simulink model "IEEE9Buses"  (R2024b)
settings: Solver=FixedStepAuto  StartTime=0  StopTime=5  FixedStep=1e-6  RelTol=1e-3
values from neighbouring files (symbols this model uses):
  SG_D_1_D = 0.01056    [SG9_parameters.m]
  SG_D_1_EnableSaturation = 0    [SG9_parameters.m]
  SG_D_1_f0 = 60    [SG9_parameters.m]
  SG_D_1_H = 7.5    [SG9_parameters.m]
  SG_D_1_K_A = 20    [SG9_parameters.m]
  SG_D_1_K_E = 1.000000e+1    (= 10)    [SG9_parameters.m]
  SG_D_1_K_F = 2.363    [SG9_parameters.m]
  SG_D_1_K_s = 5    [SG9_parameters.m]
  SG_D_1_R_a = 0.001088    [SG9_parameters.m]
  SG_D_1_S_A = 1    [SG9_parameters.m]
  SG_D_1_S_B = 0.103    [SG9_parameters.m]
  SG_D_1_S_N = 10.659857    [SG9_parameters.m]
  SG_D_1_SpeedPara = 200    [SG9_parameters.m]
  SG_D_1_T_0 = 0.720173    [SG9_parameters.m]
  SG_D_1_T_1 = 0.3    [SG9_parameters.m]
  SG_D_1_T_2 = 0.05    [SG9_parameters.m]
  SG_D_1_T_3 = 0.02    [SG9_parameters.m]
  SG_D_1_T_4 = 0.005    [SG9_parameters.m]
  SG_D_1_T_A = 0.02    [SG9_parameters.m]
  SG_D_1_T_dd = 8.000000e+0    (= 8)    [SG9_parameters.m]
  SG_D_1_T_ddd = 0.04    [SG9_parameters.m]
  SG_D_1_T_E = 0.314    [SG9_parameters.m]
  SG_D_1_T_F = 0.35    [SG9_parameters.m]
  SG_D_1_T_qd = 0.8    [SG9_parameters.m]
  SG_D_1_T_qdd = 0.02    [SG9_parameters.m]
  SG_D_1_T_speed = 0.1    [SG9_parameters.m]
  SG_D_1_T_w = 0.5    [SG9_parameters.m]
  SG_D_1_V_ref = 1.990276    [SG9_parameters.m]
  SG_D_1_w_ref = 376.991118    [SG9_parameters.m]
  SG_D_1_x_d = 1.9    [SG9_parameters.m]
  SG_D_1_x_dd = 0.302    [SG9_parameters.m]
  SG_D_1_x_ddd = 0.204    [SG9_parameters.m]
  SG_D_1_x_l = 0.05    [SG9_parameters.m]
  SG_D_1_x_q = 1.3    [SG9_parameters.m]
  SG_D_1_x_qd = 0.5    [SG9_parameters.m]
  SG_D_1_x_qdd = 0.3    [SG9_parameters.m]
  SG_D_2_D = 0.01056    [SG9_parameters.m]
  SG_D_2_EnableSaturation = 0    [SG9_parameters.m]
  SG_D_2_f0 = 60    [SG9_parameters.m]
  SG_D_2_H = 7.5    [SG9_parameters.m]
  SG_D_2_K_A = 20    [SG9_parameters.m]
  SG_D_2_K_E = 1.000000e+1    (= 10)    [SG9_parameters.m]
  SG_D_2_K_F = 2.363    [SG9_parameters.m]
  SG_D_2_K_s = 0.5    [SG9_parameters.m]
  SG_D_2_R_a = 0.001088    [SG9_parameters.m]
  SG_D_2_S_A = 1    [SG9_parameters.m]
  SG_D_2_S_B = 0.103    [SG9_parameters.m]
  SG_D_2_S_N = 10.659857    [SG9_parameters.m]
  SG_D_2_SpeedPara = 200    [SG9_parameters.m]
  SG_D_2_T_0 = 1.632913    [SG9_parameters.m]
  SG_D_2_T_1 = 0.2    [SG9_parameters.m]
  SG_D_2_T_2 = 0.05    [SG9_parameters.m]
  SG_D_2_T_3 = 0.02    [SG9_parameters.m]
  SG_D_2_T_4 = 0.005    [SG9_parameters.m]
  SG_D_2_T_A = 0.02    [SG9_parameters.m]
  SG_D_2_T_dd = 8.000000e+0    (= 8)    [SG9_parameters.m]
  SG_D_2_T_ddd = 0.04    [SG9_parameters.m]
  SG_D_2_T_E = 0.314    [SG9_parameters.m]
  SG_D_2_T_F = 0.35    [SG9_parameters.m]
  SG_D_2_T_qd = 0.8    [SG9_parameters.m]
  SG_D_2_T_qdd = 0.02    [SG9_parameters.m]
  SG_D_2_T_speed = 0.1    [SG9_parameters.m]
  SG_D_2_T_w = 0.5    [SG9_parameters.m]
  SG_D_2_V_ref = 2.662631    [SG9_parameters.m]
  SG_D_2_w_ref = 376.991118    [SG9_parameters.m]
  SG_D_2_x_d = 1.9    [SG9_parameters.m]
  SG_D_2_x_dd = 0.302    [SG9_parameters.m]
  SG_D_2_x_ddd = 0.204    [SG9_parameters.m]
  SG_D_2_x_l = 0.05    [SG9_parameters.m]
  SG_D_2_x_q = 1.3    [SG9_parameters.m]
  SG_D_2_x_qd = 0.5    [SG9_parameters.m]
  SG_D_2_x_qdd = 0.3    [SG9_parameters.m]
  SG_D_3_D = 0.01056    [SG9_parameters.m]
  SG_D_3_EnableSaturation = 0    [SG9_parameters.m]
  SG_D_3_f0 = 60    [SG9_parameters.m]
  SG_D_3_H = 7.5    [SG9_parameters.m]
  SG_D_3_K_A = 20    [SG9_parameters.m]
  SG_D_3_K_E = 1.000000e+1    (= 10)    [SG9_parameters.m]
  SG_D_3_K_F = 2.363    [SG9_parameters.m]
  SG_D_3_K_s = 0.5    [SG9_parameters.m]
  SG_D_3_R_a = 0.001088    [SG9_parameters.m]
  SG_D_3_S_A = 1    [SG9_parameters.m]
  SG_D_3_S_B = 0.103    [SG9_parameters.m]
  SG_D_3_S_N = 10.659857    [SG9_parameters.m]
  SG_D_3_SpeedPara = 200    [SG9_parameters.m]
  SG_D_3_T_0 = 0.850788    [SG9_parameters.m]
  SG_D_3_T_1 = 0.2    [SG9_parameters.m]
  SG_D_3_T_2 = 0.05    [SG9_parameters.m]
  SG_D_3_T_3 = 0.02    [SG9_parameters.m]
  SG_D_3_T_4 = 0.005    [SG9_parameters.m]
  SG_D_3_T_A = 0.02    [SG9_parameters.m]
  SG_D_3_T_dd = 8.000000e+0    (= 8)    [SG9_parameters.m]
  SG_D_3_T_ddd = 0.04    [SG9_parameters.m]
  SG_D_3_T_E = 0.314    [SG9_parameters.m]
  SG_D_3_T_F = 0.35    [SG9_parameters.m]
  SG_D_3_T_qd = 0.8    [SG9_parameters.m]
  SG_D_3_T_qdd = 0.02    [SG9_parameters.m]
  SG_D_3_T_speed = 0.1    [SG9_parameters.m]
  SG_D_3_T_w = 0.5    [SG9_parameters.m]
  SG_D_3_V_ref = 1.915682    [SG9_parameters.m]
  SG_D_3_w_ref = 376.991118    [SG9_parameters.m]
  SG_D_3_x_d = 1.9    [SG9_parameters.m]
  SG_D_3_x_dd = 0.302    [SG9_parameters.m]
  SG_D_3_x_ddd = 0.204    [SG9_parameters.m]
  SG_D_3_x_l = 0.05    [SG9_parameters.m]
  SG_D_3_x_q = 1.3    [SG9_parameters.m]
  SG_D_3_x_qd = 0.5    [SG9_parameters.m]
  SG_D_3_x_qdd = 0.3    [SG9_parameters.m]
(part 1 of 9)
settings Model: SimulationMode=accelerator  Creator=Greg  LastModifiedBy=Greg
settings DataIOCC: ReturnWorkspaceOutputs=off

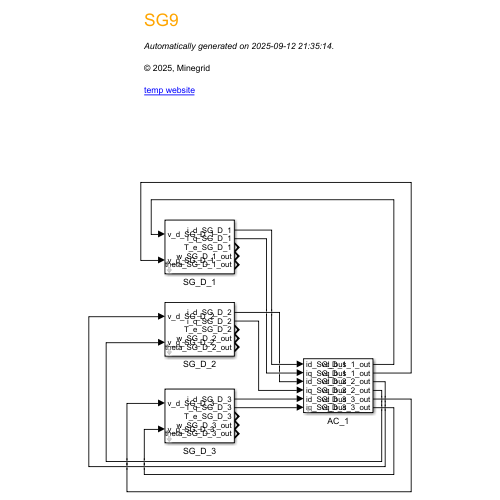
[thumbnail: Simulink's stored preview of the top-level diagram]
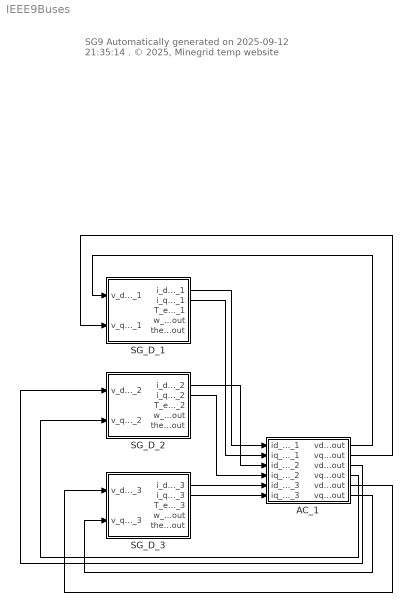
== system IEEE9Buses ==
  note: SG9
      | Automatically generated on 2025-09-12 21:35:14 .
      | © 2025, Minegrid
      | temp website
  AC_1 : Subsystem  mask(AC_1){}
      mask help: Parameters Interface of AC_1
  SG_D_1 : Subsystem  mask(SG_D_1){T_0=SG_D_1_T_0, w_ref=SG_D_1_w_ref, V_ref=SG_D_1_V_ref, x_d=SG_D_1_x_d, x_dd=SG_D_1_x_dd, x_ddd=SG_D_1_x_ddd, x_q=SG_D_1_x_q, x_qd=SG_D_1_x_qd, x_qdd=SG_D_1_x_qdd, x_l=SG_D_1_x_l, R_a=SG_D_1_R_a, T_dd=SG_D_1_T_dd, T_ddd=SG_D_1_T_ddd, T_qd=SG_D_1_T_qd, T_qdd=SG_D_1_T_qdd, H=SG_D_1_H, D=SG_D_1_D, SpeedPara=SG_D_1_SpeedPara, K_A=SG_D_1_K_A, EnableSaturation=SG_D_1_EnableSaturation, f0=SG_D_1_f0, T_speed=SG_D_1_T_speed, T_E=SG_D_1_T_E, T_A=SG_D_1_T_A, T_F=SG_D_1_T_F, K_E=SG_D_1_K_E, K_F=SG_D_1_K_F, K_s=SG_D_1_K_s, T_1=SG_D_1_T_1, T_2=SG_D_1_T_2, T_3=SG_D_1_T_3, T_4=SG_D_1_T_4, T_w=SG_D_1_T_w, S_A=SG_D_1_S_A, S_B=SG_D_1_S_B, S_N=SG_D_1_S_N}
      mask help: Parameters Interface of SG_D_1
  SG_D_2 : Subsystem  mask(SG_D_2){T_0=SG_D_2_T_0, w_ref=SG_D_2_w_ref, V_ref=SG_D_2_V_ref, x_d=SG_D_2_x_d, x_dd=SG_D_2_x_dd, x_ddd=SG_D_2_x_ddd, x_q=SG_D_2_x_q, x_qd=SG_D_2_x_qd, x_qdd=SG_D_2_x_qdd, x_l=SG_D_2_x_l, R_a=SG_D_2_R_a, T_dd=SG_D_2_T_dd, T_ddd=SG_D_2_T_ddd, T_qd=SG_D_2_T_qd, T_qdd=SG_D_2_T_qdd, H=SG_D_2_H, D=SG_D_2_D, SpeedPara=SG_D_2_SpeedPara, K_A=SG_D_2_K_A, EnableSaturation=SG_D_2_EnableSaturation, f0=SG_D_2_f0, T_speed=SG_D_2_T_speed, T_E=SG_D_2_T_E, T_A=SG_D_2_T_A, T_F=SG_D_2_T_F, K_E=SG_D_2_K_E, K_F=SG_D_2_K_F, K_s=SG_D_2_K_s, T_1=SG_D_2_T_1, T_2=SG_D_2_T_2, T_3=SG_D_2_T_3, T_4=SG_D_2_T_4, T_w=SG_D_2_T_w, S_A=SG_D_2_S_A, S_B=SG_D_2_S_B, S_N=SG_D_2_S_N}
      mask help: Parameters Interface of SG_D_2
  SG_D_3 : Subsystem  mask(SG_D_3){T_0=SG_D_3_T_0, w_ref=SG_D_3_w_ref, V_ref=SG_D_3_V_ref, x_d=SG_D_3_x_d, x_dd=SG_D_3_x_dd, x_ddd=SG_D_3_x_ddd, x_q=SG_D_3_x_q, x_qd=SG_D_3_x_qd, x_qdd=SG_D_3_x_qdd, x_l=SG_D_3_x_l, R_a=SG_D_3_R_a, T_dd=SG_D_3_T_dd, T_ddd=SG_D_3_T_ddd, T_qd=SG_D_3_T_qd, T_qdd=SG_D_3_T_qdd, H=SG_D_3_H, D=SG_D_3_D, SpeedPara=SG_D_3_SpeedPara, K_A=SG_D_3_K_A, EnableSaturation=SG_D_3_EnableSaturation, f0=SG_D_3_f0, T_speed=SG_D_3_T_speed, T_E=SG_D_3_T_E, T_A=SG_D_3_T_A, T_F=SG_D_3_T_F, K_E=SG_D_3_K_E, K_F=SG_D_3_K_F, K_s=SG_D_3_K_s, T_1=SG_D_3_T_1, T_2=SG_D_3_T_2, T_3=SG_D_3_T_3, T_4=SG_D_3_T_4, T_w=SG_D_3_T_w, S_A=SG_D_3_S_A, S_B=SG_D_3_S_B, S_N=SG_D_3_S_N}
      mask help: Parameters Interface of SG_D_3
  wires:
  SG_D_2/2(i_q_SG_D_2) -> AC_1/4(iq_SG_D_2)
  SG_D_1/2(i_q_SG_D_1) -> AC_1/2(iq_SG_D_1)
  SG_D_1/1(i_d_SG_D_1) -> AC_1/1(id_SG_D_1)
  SG_D_2/1(i_d_SG_D_2) -> AC_1/3(id_SG_D_2)
  AC_1/1(vd_bus_1_out) -> SG_D_1/1(v_d_SG_D_1)
  SG_D_3/1(i_d_SG_D_3) -> AC_1/5(id_SG_D_3)
  AC_1/2(vq_bus_1_out) -> SG_D_1/2(v_q_SG_D_1)
  SG_D_3/2(i_q_SG_D_3) -> AC_1/6(iq_SG_D_3)
  AC_1/3(vd_bus_2_out) -> SG_D_2/1(v_d_SG_D_2)
  AC_1/4(vq_bus_2_out) -> SG_D_2/2(v_q_SG_D_2)
  AC_1/5(vd_bus_3_out) -> SG_D_3/1(v_d_SG_D_3)
  AC_1/6(vq_bus_3_out) -> SG_D_3/2(v_q_SG_D_3)

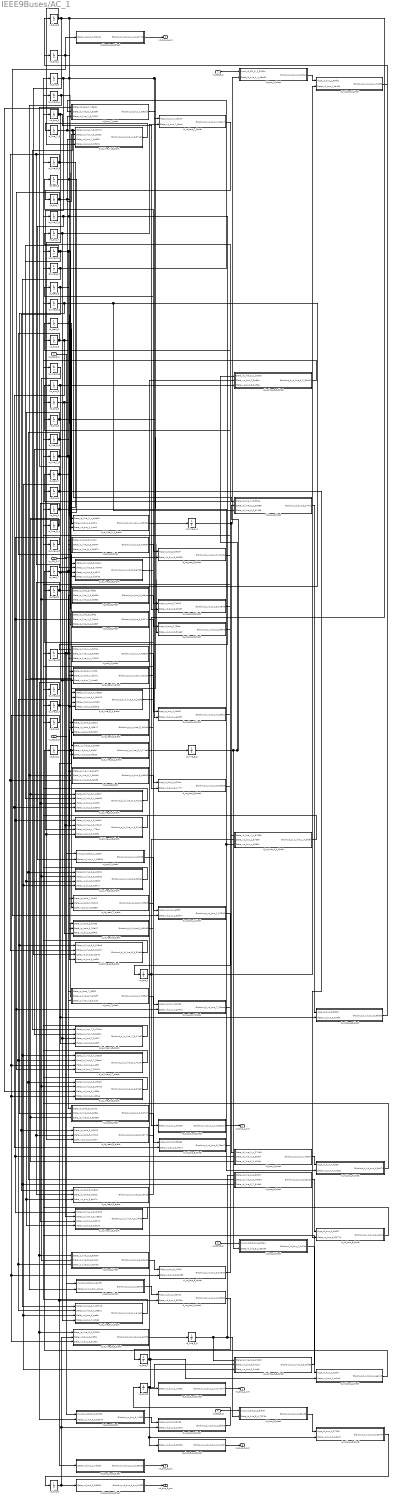
== system IEEE9Buses/AC_1 ==
  id_SG_D_1 : Inport
  iq_SG_D_1 : Inport  Port=2
  id_SG_D_2 : Inport  Port=3
  iq_SG_D_2 : Inport  Port=4
  id_SG_D_3 : Inport  Port=5
  iq_SG_D_3 : Inport  Port=6
  d_id_line_1_4_block : Subsystem
  d_id_line_3_6_block : Subsystem
  d_id_line_4_5_block : Subsystem
  d_id_line_5_6_block : Subsystem
  d_id_line_6_7_block : Subsystem
  d_id_line_7_8_block : Subsystem
  d_id_line_8_2_block : Subsystem
  d_id_line_8_9_block : Subsystem
  d_id_line_9_4_block : Subsystem
  d_id_load_5_block : Subsystem
  d_id_load_7_block : Subsystem
  d_id_load_9_block : Subsystem
  d_iq_line_1_4_block : Subsystem
  d_iq_line_3_6_block : Subsystem
  d_iq_line_4_5_block : Subsystem
  d_iq_line_5_6_block : Subsystem
  d_iq_line_6_7_block : Subsystem
  d_iq_line_7_8_block : Subsystem
  d_iq_line_8_2_block : Subsystem
  d_iq_line_8_9_block : Subsystem
  d_iq_line_9_4_block : Subsystem
  d_iq_load_5_block : Subsystem
  d_iq_load_7_block : Subsystem
  d_iq_load_9_block : Subsystem
  d_vd_bus_1_block : Subsystem
  d_vd_bus_2_block : Subsystem
  d_vd_bus_3_block : Subsystem
  d_vd_bus_4_block : Subsystem
  d_vd_bus_5_block : Subsystem
  d_vd_bus_6_block : Subsystem
  d_vd_bus_7_block : Subsystem
  d_vd_bus_8_block : Subsystem
  d_vd_bus_9_block : Subsystem
  d_vq_bus_1_block : Subsystem
  d_vq_bus_2_block : Subsystem
  d_vq_bus_3_block : Subsystem
  d_vq_bus_4_block : Subsystem
  d_vq_bus_5_block : Subsystem
  d_vq_bus_6_block : Subsystem
  d_vq_bus_7_block : Subsystem
  d_vq_bus_8_block : Subsystem
  d_vq_bus_9_block : Subsystem
  id_bus_1_block : Subsystem
  id_bus_2_block : Subsystem
  id_bus_3_block : Subsystem
  id_bus_4_block : Subsystem
  id_bus_5_block : Subsystem
  id_bus_6_block : Subsystem
  id_bus_7_block : Subsystem
  id_bus_8_block : Subsystem
  id_bus_9_block : Subsystem
  id_line_1_4 : Integrator  InitialCondition=0.7195
  id_line_3_6 : Integrator  InitialCondition=0.844
  id_line_4_5 : Integrator  InitialCondition=0.308
  id_line_5_6 : Integrator  InitialCondition=-0.6084
  id_line_6_7 : Integrator  InitialCondition=0.2452
  id_line_7_8 : Integrator  InitialCondition=-0.7713
  id_line_8_2 : Integrator  InitialCondition=-1.6311
  id_line_8_9 : Integrator  InitialCondition=0.8749
  id_line_9_4 : Integrator  InitialCondition=-0.4046
  id_load_5 : Integrator  InitialCondition=0.898817607082261
  id_load_7 : Integrator  InitialCondition=1.0183565162188208
  id_load_9 : Integrator  InitialCondition=1.2619557605717109
  iq_bus_1_block : Subsystem
  iq_bus_2_block : Subsystem
  iq_bus_3_block : Subsystem
  iq_bus_4_block : Subsystem
  iq_bus_5_block : Subsystem
  iq_bus_6_block : Subsystem
  iq_bus_7_block : Subsystem
  iq_bus_8_block : Subsystem
  iq_bus_9_block : Subsystem
  iq_line_1_4 : Integrator  InitialCondition=-0.2407
  iq_line_3_6 : Integrator  InitialCondition=0.1071
  iq_line_4_5 : Integrator  InitialCondition=-0.085
  iq_line_5_6 : Integrator  InitialCondition=0.0353
  iq_line_6_7 : Integrator  InitialCondition=-0.1419
  iq_line_7_8 : Integrator  InitialCondition=0.0257
  iq_line_8_2 : Integrator  InitialCondition=-0.1312
  iq_line_8_9 : Integrator  InitialCondition=-0.0692
  iq_line_9_4 : Integrator  InitialCondition=0.3203
  iq_load_5 : Integrator  InitialCondition=-0.37142447893959263
  iq_load_7 : Integrator  InitialCondition=-0.34407079769452764
  iq_load_9 : Integrator  InitialCondition=-0.6196286093512099
  vd_bus_1 : Integrator  InitialCondition=1.0
  vd_bus_1_out_block : Subsystem
  vd_bus_2 : Integrator  InitialCondition=0.9857952451733694
  vd_bus_2_out_block : Subsystem
  vd_bus_3 : Integrator  InitialCondition=0.9965349784480291
  vd_bus_3_out_block : Subsystem
  vd_bus_4 : Integrator  InitialCondition=0.9861362779327475
  vd_bus_5 : Integrator  InitialCondition=0.9730754311923555
  vd_bus_6 : Integrator  InitialCondition=1.0028088352065478
  vd_bus_7 : Integrator  InitialCondition=0.9855868856760395
  vd_bus_8 : Integrator  InitialCondition=0.9939961188157862
  vd_bus_9 : Integrator  InitialCondition=0.9548625268660215
  vq_bus_1 : Integrator  InitialCondition=0.0
  vq_bus_1_out_block : Subsystem
  vq_bus_2 : Integrator  InitialCondition=0.16795158407581826
  vq_bus_2_out_block : Subsystem
  vq_bus_3 : Integrator  InitialCondition=0.08317473612573835
  vq_bus_3_out_block : Subsystem
  vq_bus_4 : Integrator  InitialCondition=-0.04144590802322367
  vq_bus_5 : Integrator  InitialCondition=-0.06833870911689703
  vq_bus_6 : Integrator  InitialCondition=0.03371518392178962
  vq_bus_7 : Integrator  InitialCondition=0.01069206498389038
  vq_bus_8 : Integrator  InitialCondition=0.06600581865802534
  vq_bus_9 : Integrator  InitialCondition=-0.07263340166698863
  vd_bus_1_out : Outport
  vq_bus_1_out : Outport  Port=2
  vd_bus_2_out : Outport  Port=3
  vq_bus_2_out : Outport  Port=4
  vd_bus_3_out : Outport  Port=5
  vq_bus_3_out : Outport  Port=6
  wires:
  d_vd_bus_8_block/1(Blockout_d_vd_bus_8_9b000) -> vd_bus_8/1
  iq_bus_2_block/1(Blockout_iq_bus_2_e5997) -> d_vq_bus_2_block/1(Alge_iq_bus_2_d512d)
  vd_bus_6/1 -> d_vq_bus_6_block/2(State_vd_bus_6_b0c85), d_id_line_3_6_block/3(State_vd_bus_6_a239d), d_id_line_5_6_block/4(State_vd_bus_6_469ee), d_id_line_6_7_block/3(State_vd_bus_6_443fc)
  iq_bus_9_block/1(Blockout_iq_bus_9_40080) -> d_vq_bus_9_block/1(Alge_iq_bus_9_d9c5f)
  id_bus_3_block/1(Blockout_id_bus_3_8623b) -> d_vd_bus_3_block/1(Alge_id_bus_3_37259)
  id_bus_8_block/1(Blockout_id_bus_8_27f10) -> d_vd_bus_8_block/1(Alge_id_bus_8_fc0d0)
  d_id_line_1_4_block/1(Blockout_d_id_line_1_4_93c8d) -> id_line_1_4/1
  vq_bus_2_out_block/1(Blockout_vq_bus_2_out_74947) -> vq_bus_2_out/1
  iq_SG_D_3/1 -> iq_bus_3_block/1(Input_iq_SG_D_3_d199a)
  vd_bus_3_out_block/1(Blockout_vd_bus_3_out_02f53) -> vd_bus_3_out/1
  d_iq_line_8_2_block/1(Blockout_d_iq_line_8_2_3b9b1) -> iq_line_8_2/1
  d_vd_bus_4_block/1(Blockout_d_vd_bus_4_3a074) -> vd_bus_4/1
  id_SG_D_3/1 -> id_bus_3_block/1(Input_id_SG_D_3_5cb67)
  id_SG_D_2/1 -> id_bus_2_block/1(Input_id_SG_D_2_e59e4)
  iq_SG_D_2/1 -> iq_bus_2_block/1(Input_iq_SG_D_2_644f3)
  iq_SG_D_1/1 -> iq_bus_1_block/1(Input_iq_SG_D_1_ca28f)
  id_bus_9_block/1(Blockout_id_bus_9_52737) -> d_vd_bus_9_block/1(Alge_id_bus_9_59e86)
  d_vd_bus_3_block/1(Blockout_d_vd_bus_3_60d94) -> vd_bus_3/1
  vq_bus_9/1 -> d_vd_bus_9_block/2(State_vq_bus_9_f7872), d_iq_line_9_4_block/4(State_vq_bus_9_ae56d), d_iq_load_9_block/3(State_vq_bus_9_5d2b3), d_iq_line_8_9_block/4(State_vq_bus_9_bbb4a)
  d_vq_bus_6_block/1(Blockout_d_vq_bus_6_6730a) -> vq_bus_6/1
  id_SG_D_1/1 -> id_bus_1_block/1(Input_id_SG_D_1_3262c)
  d_id_line_3_6_block/1(Blockout_d_id_line_3_6_e09c3) -> id_line_3_6/1
  d_vq_bus_5_block/1(Blockout_d_vq_bus_5_a48d8) -> vq_bus_5/1
  vq_bus_3_out_block/1(Blockout_vq_bus_3_out_11dc3) -> vq_bus_3_out/1
  iq_bus_8_block/1(Blockout_iq_bus_8_e3563) -> d_vq_bus_8_block/1(Alge_iq_bus_8_c37e6)
  iq_bus_7_block/1(Blockout_iq_bus_7_33867) -> d_vq_bus_7_block/1(Alge_iq_bus_7_d2b8e)
  vd_bus_1/1 -> d_id_line_1_4_block/2(State_vd_bus_1_adf11), vd_bus_1_out_block/1(State_vd_bus_1_30b4d), d_vq_bus_1_block/2(State_vd_bus_1_09d77)
  iq_line_8_9/1 -> d_id_line_8_9_block/2(State_iq_line_8_9_9c429), iq_bus_8_block/3(State_iq_line_8_9_ce938), d_iq_line_8_9_block/2(State_iq_line_8_9_4d480), iq_bus_9_block/2(State_iq_line_8_9_c4804)
  id_bus_7_block/1(Blockout_id_bus_7_881bd) -> d_vd_bus_7_block/1(Alge_id_bus_7_c3139)
  id_bus_5_block/1(Blockout_id_bus_5_5017c) -> d_vd_bus_5_block/1(Alge_id_bus_5_7f9ce)
  iq_bus_6_block/1(Blockout_iq_bus_6_e51e3) -> d_vq_bus_6_block/1(Alge_iq_bus_6_c7a6f)
  d_id_load_7_block/1(Blockout_d_id_load_7_5535f) -> id_load_7/1
  vd_bus_7/1 -> d_id_load_7_block/3(State_vd_bus_7_a9ee9), d_id_line_7_8_block/3(State_vd_bus_7_ec582), d_vq_bus_7_block/2(State_vd_bus_7_25076), d_id_line_6_7_block/4(State_vd_bus_7_82461)
  d_id_load_9_block/1(Blockout_d_id_load_9_d90d0) -> id_load_9/1
  id_line_8_9/1 -> d_id_line_8_9_block/1(State_id_line_8_9_b15e6), id_bus_9_block/2(State_id_line_8_9_2ef8e), id_bus_8_block/3(State_id_line_8_9_87c38), d_iq_line_8_9_block/1(State_id_line_8_9_9ac4c)
  iq_line_6_7/1 -> iq_bus_6_block/3(State_iq_line_6_7_0570d), d_iq_line_6_7_block/2(State_iq_line_6_7_68911), d_id_line_6_7_block/2(State_iq_line_6_7_95ec9), iq_bus_7_block/2(State_iq_line_6_7_a92f3)
  id_line_4_5/1 -> d_iq_line_4_5_block/1(State_id_line_4_5_bb2d8), id_bus_4_block/2(State_id_line_4_5_666cf), d_id_line_4_5_block/1(State_id_line_4_5_9d9bf), id_bus_5_block/2(State_id_line_4_5_7fba6)
  id_bus_6_block/1(Blockout_id_bus_6_b82c2) -> d_vd_bus_6_block/1(Alge_id_bus_6_00f20)
  iq_bus_5_block/1(Blockout_iq_bus_5_cd3aa) -> d_vq_bus_5_block/1(Alge_iq_bus_5_7cd16)
  id_bus_2_block/1(Blockout_id_bus_2_0c7b0) -> d_vd_bus_2_block/1(Alge_id_bus_2_43cf4)
  id_line_6_7/1 -> id_bus_6_block/3(State_id_line_6_7_545c3), d_iq_line_6_7_block/1(State_id_line_6_7_95748), d_id_line_6_7_block/1(State_id_line_6_7_a6336), id_bus_7_block/2(State_id_line_6_7_e269f)
  iq_bus_4_block/1(Blockout_iq_bus_4_66e6a) -> d_vq_bus_4_block/1(Alge_iq_bus_4_4be37)
  d_vq_bus_9_block/1(Blockout_d_vq_bus_9_7a2cb) -> vq_bus_9/1
  iq_line_9_4/1 -> iq_bus_4_block/3(State_iq_line_9_4_7b513), iq_bus_9_block/3(State_iq_line_9_4_0e87b), d_iq_line_9_4_block/2(State_iq_line_9_4_5ae9b), d_id_line_9_4_block/2(State_iq_line_9_4_9b423)
  vq_bus_6/1 -> d_iq_line_6_7_block/3(State_vq_bus_6_aeffa), d_iq_line_3_6_block/3(State_vq_bus_6_14cd6), d_iq_line_5_6_block/4(State_vq_bus_6_e6417), d_vd_bus_6_block/2(State_vq_bus_6_6b77a)
  id_load_5/1 -> d_iq_load_5_block/1(State_id_load_5_3469a), d_id_load_5_block/1(State_id_load_5_6942d), id_bus_5_block/1(State_id_load_5_1fb8c)
  iq_bus_3_block/1(Blockout_iq_bus_3_7a5f4) -> d_vq_bus_3_block/1(Alge_iq_bus_3_4618e)
  id_line_5_6/1 -> d_id_line_5_6_block/1(State_id_line_5_6_30ca9), id_bus_6_block/2(State_id_line_5_6_48a69), d_iq_line_5_6_block/1(State_id_line_5_6_bb5d1), id_bus_5_block/3(State_id_line_5_6_0d80f)
  id_bus_4_block/1(Blockout_id_bus_4_7eb34) -> d_vd_bus_4_block/1(Alge_id_bus_4_fcb80)
  vd_bus_1_out_block/1(Blockout_vd_bus_1_out_0277b) -> vd_bus_1_out/1
  vq_bus_1_out_block/1(Blockout_vq_bus_1_out_8292c) -> vq_bus_1_out/1
  id_line_9_4/1 -> id_bus_4_block/3(State_id_line_9_4_46c2c), id_bus_9_block/3(State_id_line_9_4_80368), d_iq_line_9_4_block/1(State_id_line_9_4_069c7), d_id_line_9_4_block/1(State_id_line_9_4_75390)
  iq_line_8_2/1 -> iq_bus_2_block/2(State_iq_line_8_2_4a7a6), iq_bus_8_block/2(State_iq_line_8_2_9e1b5), d_id_line_8_2_block/1(State_iq_line_8_2_d048e)
  iq_bus_1_block/1(Blockout_iq_bus_1_b29d9) -> d_vq_bus_1_block/1(Alge_iq_bus_1_ef3c8)
  id_bus_1_block/1(Blockout_id_bus_1_d304c) -> d_vd_bus_1_block/1(Alge_id_bus_1_5efe2)
  vd_bus_2_out_block/1(Blockout_vd_bus_2_out_05523) -> vd_bus_2_out/1
  d_id_line_8_2_block/1(Blockout_d_id_line_8_2_17ce9) -> id_line_8_2/1
  vq_bus_5/1 -> d_iq_load_5_block/3(State_vq_bus_5_8a47c), d_iq_line_4_5_block/4(State_vq_bus_5_6d109), d_iq_line_5_6_block/3(State_vq_bus_5_5a835), d_vd_bus_5_block/2(State_vq_bus_5_81ea0)
  d_id_line_9_4_block/1(Blockout_d_id_line_9_4_bcdf8) -> id_line_9_4/1
  vd_bus_8/1 -> d_vq_bus_8_block/2(State_vd_bus_8_17777), d_id_line_8_2_block/3(State_vd_bus_8_4faee), d_id_line_8_9_block/3(State_vd_bus_8_2da45), d_id_line_7_8_block/4(State_vd_bus_8_932d1)
  iq_load_5/1 -> d_iq_load_5_block/2(State_iq_load_5_30dc2), d_id_load_5_block/2(State_iq_load_5_374bd), iq_bus_5_block/1(State_iq_load_5_4f98c)
  id_load_7/1 -> d_iq_load_7_block/1(State_id_load_7_27cc0), d_id_load_7_block/1(State_id_load_7_9c11f), id_bus_7_block/1(State_id_load_7_766eb)
  id_line_8_2/1 -> d_iq_line_8_2_block/1(State_id_line_8_2_1a8da), id_bus_8_block/2(State_id_line_8_2_3b688), id_bus_2_block/2(State_id_line_8_2_6326a)
  id_line_3_6/1 -> id_bus_3_block/2(State_id_line_3_6_7876d), id_bus_6_block/1(State_id_line_3_6_8987c), d_iq_line_3_6_block/1(State_id_line_3_6_232a9)
  iq_line_7_8/1 -> iq_bus_7_block/3(State_iq_line_7_8_2c1c0), iq_bus_8_block/1(State_iq_line_7_8_aee75), d_id_line_7_8_block/2(State_iq_line_7_8_ca362), d_iq_line_7_8_block/2(State_iq_line_7_8_5efa1)
  id_line_7_8/1 -> d_id_line_7_8_block/1(State_id_line_7_8_3b707), d_iq_line_7_8_block/1(State_id_line_7_8_521a4), id_bus_8_block/1(State_id_line_7_8_ffd1a), id_bus_7_block/3(State_id_line_7_8_76347)
  vd_bus_2/1 -> d_vq_bus_2_block/2(State_vd_bus_2_9829a), vd_bus_2_out_block/1(State_vd_bus_2_7ad9e), d_id_line_8_2_block/2(State_vd_bus_2_bbfdf)
  iq_line_3_6/1 -> d_id_line_3_6_block/1(State_iq_line_3_6_282d0), iq_bus_3_block/2(State_iq_line_3_6_8aa40), iq_bus_6_block/1(State_iq_line_3_6_58a90)
  iq_line_5_6/1 -> d_id_line_5_6_block/2(State_iq_line_5_6_587be), iq_bus_6_block/2(State_iq_line_5_6_012cd), d_iq_line_5_6_block/2(State_iq_line_5_6_03d26), iq_bus_5_block/3(State_iq_line_5_6_de832)
  iq_line_4_5/1 -> d_id_line_4_5_block/2(State_iq_line_4_5_254e7), d_iq_line_4_5_block/2(State_iq_line_4_5_78e2b), iq_bus_4_block/2(State_iq_line_4_5_eba88), iq_bus_5_block/2(State_iq_line_4_5_8b006)
  iq_load_7/1 -> d_id_load_7_block/2(State_iq_load_7_51219), d_iq_load_7_block/2(State_iq_load_7_db75c), iq_bus_7_block/1(State_iq_load_7_0f831)
  id_line_1_4/1 -> id_bus_1_block/2(State_id_line_1_4_5eb51), id_bus_4_block/1(State_id_line_1_4_271d8), d_iq_line_1_4_block/1(State_id_line_1_4_57d80)
  vq_bus_4/1 -> d_iq_line_1_4_block/3(State_vq_bus_4_b5984), d_vd_bus_4_block/2(State_vq_bus_4_57d81), d_iq_line_9_4_block/3(State_vq_bus_4_81c39), d_iq_line_4_5_block/3(State_vq_bus_4_a5b76)
  iq_line_1_4/1 -> d_id_line_1_4_block/1(State_iq_line_1_4_a5e26), iq_bus_4_block/1(State_iq_line_1_4_f419e), iq_bus_1_block/2(State_iq_line_1_4_8883d)
  vd_bus_4/1 -> d_vq_bus_4_block/2(State_vd_bus_4_edd2f), d_id_line_9_4_block/3(State_vd_bus_4_e2c56), d_id_line_1_4_block/3(State_vd_bus_4_44d4f), d_id_line_4_5_block/3(State_vd_bus_4_779cd)
  iq_load_9/1 -> d_id_load_9_block/2(State_iq_load_9_20a57), d_iq_load_9_block/2(State_iq_load_9_d6a72), iq_bus_9_block/1(State_iq_load_9_c7d1b)
  vq_bus_1/1 -> d_vd_bus_1_block/2(State_vq_bus_1_fa40c), d_iq_line_1_4_block/2(State_vq_bus_1_b7ee6), vq_bus_1_out_block/1(State_vq_bus_1_02b5e)
  id_load_9/1 -> d_id_load_9_block/1(State_id_load_9_f793a), d_iq_load_9_block/1(State_id_load_9_2692c), id_bus_9_block/1(State_id_load_9_21730)
  vd_bus_5/1 -> d_id_line_4_5_block/4(State_vd_bus_5_5d0f4), d_id_load_5_block/3(State_vd_bus_5_7ebb7), d_vq_bus_5_block/2(State_vd_bus_5_232bf), d_id_line_5_6_block/3(State_vd_bus_5_135fa)
  vd_bus_9/1 -> d_id_line_8_9_block/4(State_vd_bus_9_bcf84), d_id_line_9_4_block/4(State_vd_bus_9_f9bbb), d_vq_bus_9_block/2(State_vd_bus_9_b3036), d_id_load_9_block/3(State_vd_bus_9_d8fb5)
  vq_bus_8/1 -> d_vd_bus_8_block/2(State_vq_bus_8_879f9), d_iq_line_7_8_block/4(State_vq_bus_8_ca51f), d_iq_line_8_9_block/3(State_vq_bus_8_a4521), d_iq_line_8_2_block/3(State_vq_bus_8_54d3e)
  vq_bus_7/1 -> d_iq_line_6_7_block/4(State_vq_bus_7_cc662), d_iq_line_7_8_block/3(State_vq_bus_7_5101f), d_iq_load_7_block/3(State_vq_bus_7_44ad8), d_vd_bus_7_block/2(State_vq_bus_7_fddcc)
  vd_bus_3/1 -> d_vq_bus_3_block/2(State_vd_bus_3_13373), d_id_line_3_6_block/2(State_vd_bus_3_4df94), vd_bus_3_out_block/1(State_vd_bus_3_69656)
  vq_bus_3/1 -> d_vd_bus_3_block/2(State_vq_bus_3_a84ef), vq_bus_3_out_block/1(State_vq_bus_3_9203b), d_iq_line_3_6_block/2(State_vq_bus_3_b412d)
  vq_bus_2/1 -> d_vd_bus_2_block/2(State_vq_bus_2_cc1ad), vq_bus_2_out_block/1(State_vq_bus_2_14eae), d_iq_line_8_2_block/2(State_vq_bus_2_6a8ad)
  d_vq_bus_1_block/1(Blockout_d_vq_bus_1_67500) -> vq_bus_1/1
  d_id_line_7_8_block/1(Blockout_d_id_line_7_8_9746d) -> id_line_7_8/1
  d_id_line_6_7_block/1(Blockout_d_id_line_6_7_75140) -> id_line_6_7/1
  d_iq_line_6_7_block/1(Blockout_d_iq_line_6_7_a4a1a) -> iq_line_6_7/1
  d_iq_load_5_block/1(Blockout_d_iq_load_5_26519) -> iq_load_5/1
  d_id_line_5_6_block/1(Blockout_d_id_line_5_6_0d6a1) -> id_line_5_6/1
  d_id_line_4_5_block/1(Blockout_d_id_line_4_5_01c13) -> id_line_4_5/1
  d_id_line_8_9_block/1(Blockout_d_id_line_8_9_50e3a) -> id_line_8_9/1
  d_vq_bus_3_block/1(Blockout_d_vq_bus_3_efd63) -> vq_bus_3/1
  d_id_load_5_block/1(Blockout_d_id_load_5_1877c) -> id_load_5/1
  d_vq_bus_4_block/1(Blockout_d_vq_bus_4_2eed2) -> vq_bus_4/1
  d_iq_line_1_4_block/1(Blockout_d_iq_line_1_4_afc5f) -> iq_line_1_4/1
  d_iq_line_3_6_block/1(Blockout_d_iq_line_3_6_9df33) -> iq_line_3_6/1
  d_vq_bus_7_block/1(Blockout_d_vq_bus_7_29dea) -> vq_bus_7/1
  d_iq_line_4_5_block/1(Blockout_d_iq_line_4_5_7f0d8) -> iq_line_4_5/1
  d_iq_line_5_6_block/1(Blockout_d_iq_line_5_6_f65e1) -> iq_line_5_6/1
  d_iq_load_9_block/1(Blockout_d_iq_load_9_040c9) -> iq_load_9/1
  d_iq_line_7_8_block/1(Blockout_d_iq_line_7_8_47c62) -> iq_line_7_8/1
  d_vd_bus_2_block/1(Blockout_d_vd_bus_2_ea113) -> vd_bus_2/1
  d_iq_line_8_9_block/1(Blockout_d_iq_line_8_9_a326a) -> iq_line_8_9/1
  d_iq_line_9_4_block/1(Blockout_d_iq_line_9_4_42bd3) -> iq_line_9_4/1
  d_iq_load_7_block/1(Blockout_d_iq_load_7_b1dc5) -> iq_load_7/1
  d_vq_bus_8_block/1(Blockout_d_vq_bus_8_0c63e) -> vq_bus_8/1
  d_vd_bus_1_block/1(Blockout_d_vd_bus_1_31f38) -> vd_bus_1/1
  d_vd_bus_9_block/1(Blockout_d_vd_bus_9_33aa7) -> vd_bus_9/1
  d_vd_bus_5_block/1(Blockout_d_vd_bus_5_ffea6) -> vd_bus_5/1
  d_vd_bus_7_block/1(Blockout_d_vd_bus_7_02e17) -> vd_bus_7/1
  d_vd_bus_6_block/1(Blockout_d_vd_bus_6_a81cc) -> vd_bus_6/1
  d_vq_bus_2_block/1(Blockout_d_vq_bus_2_b988a) -> vq_bus_2/1

== system IEEE9Buses/SG_D_1 ==
  v_d_SG_D_1 : Inport
  v_q_SG_D_1 : Inport  Port=2
  E_fd_SG_D_1 : Integrator  InitialCondition=1.9805513012329263
  Px_1_SG_D_1 : Integrator  InitialCondition=0.0
  Px_2_SG_D_1 : Integrator  InitialCondition=0.0
  Px_3_SG_D_1 : Integrator  InitialCondition=1.3587350977693559e-31
  R_f_SG_D_1 : Integrator  InitialCondition=13.371550642324015
  T_e_SG_D_1_block : Subsystem
  T_m_SG_D_1 : Integrator  InitialCondition=0.7201733550664303
  V_f_SG_D_1 : Integrator  InitialCondition=19.805513012329264
  d_E_fd_SG_D_1_block : Subsystem
  d_Px_1_SG_D_1_block : Subsystem
  d_Px_2_SG_D_1_block : Subsystem
  d_Px_3_SG_D_1_block : Subsystem
  d_R_f_SG_D_1_block : Subsystem
  d_T_m_SG_D_1_block : Subsystem
  d_V_f_SG_D_1_block : Subsystem
  d_psi_1d_SG_D_1_block : Subsystem
  d_psi_d_SG_D_1_block : Subsystem
  d_psi_fd_SG_D_1_block : Subsystem
  d_psi_gq_SG_D_1_block : Subsystem
  d_psi_kq_SG_D_1_block : Subsystem
  d_psi_q_SG_D_1_block : Subsystem
  d_theta_SG_D_1_block : Subsystem
  d_w_SG_D_1_block : Subsystem
  i_d_SG_D_1_block : Subsystem
  i_q_SG_D_1_block : Subsystem
  psi_1d_SG_D_1 : Integrator  InitialCondition=0.845823229911384
  psi_d_SG_D_1 : Integrator  InitialCondition=0.8151549036594502
  psi_fd_SG_D_1 : Integrator  InitialCondition=1.0003915942211292
  psi_gq_SG_D_1 : Integrator  InitialCondition=0.35728835356649113
  psi_kq_SG_D_1 : Integrator  InitialCondition=-0.5582630524476424
  psi_q_SG_D_1 : Integrator  InitialCondition=-0.580593574545548
  theta_SG_D_1 : Integrator  InitialCondition=0.6186381378069596
  theta_SG_D_1_out_block : Subsystem
  w_SG_D_1 : Integrator  InitialCondition=376.99111843077515
  w_SG_D_1_out_block : Subsystem
  i_d_SG_D_1 : Outport
  i_q_SG_D_1 : Outport  Port=2
  T_e_SG_D_1 : Outport  Port=3
  w_SG_D_1_out : Outport  Port=4
  theta_SG_D_1_out : Outport  Port=5
  wires:
  d_Px_1_SG_D_1_block/1(Blockout_d_Px_1_SG_D_1_cf474) -> Px_1_SG_D_1/1
  V_f_SG_D_1/1 -> d_V_f_SG_D_1_block/14(State_V_f_SG_D_1_8970f), d_E_fd_SG_D_1_block/2(State_V_f_SG_D_1_23896)
  psi_kq_SG_D_1/1 -> d_psi_q_SG_D_1_block/2(State_psi_kq_SG_D_1_3d8c9), d_V_f_SG_D_1_block/10(State_psi_kq_SG_D_1_48f93), d_w_SG_D_1_block/5(State_psi_kq_SG_D_1_49621), i_d_SG_D_1_block/2(State_psi_kq_SG_D_1_e3ffd), i_q_SG_D_1_block/2(State_psi_kq_SG_D_1_bbf34), d_psi_kq_SG_D_1_block/4(State_psi_kq_SG_D_1_6f435), d_psi_kq_SG_D_1_block/2(State_psi_kq_SG_D_1_2245f), d_psi_gq_SG_D_1_block/3(State_psi_kq_SG_D_1_536d2), d_psi_gq_SG_D_1_block/5(State_psi_kq_SG_D_1_a18e9), d_psi_gq_SG_D_1_block/8(State_psi_kq_SG_D_1_64214), T_e_SG_D_1_block/3(State_psi_kq_SG_D_1_b55ca)
  w_SG_D_1_out_block/1(Blockout_w_SG_D_1_out_88950) -> w_SG_D_1_out/1
  d_theta_SG_D_1_block/1(Blockout_d_theta_SG_D_1_2b5f4) -> theta_SG_D_1/1
  w_SG_D_1/1 -> d_Px_2_SG_D_1_block/4(State_w_SG_D_1_fc7e0), d_Px_1_SG_D_1_block/2(State_w_SG_D_1_abb95), d_psi_d_SG_D_1_block/9(State_w_SG_D_1_13bdb), d_w_SG_D_1_block/1(State_w_SG_D_1_f41ee), d_T_m_SG_D_1_block/1(State_w_SG_D_1_aacae), d_V_f_SG_D_1_block/8(State_w_SG_D_1_1fa23), d_theta_SG_D_1_block/1(State_w_SG_D_1_e3939), d_V_f_SG_D_1_block/13(State_w_SG_D_1_ee92d), d_psi_q_SG_D_1_block/9(State_w_SG_D_1_4a22e), w_SG_D_1_out_block/1(State_w_SG_D_1_1a398), d_Px_3_SG_D_1_block/6(State_w_SG_D_1_841ae)
  d_Px_3_SG_D_1_block/1(Blockout_d_Px_3_SG_D_1_5e87f) -> Px_3_SG_D_1/1
  d_T_m_SG_D_1_block/1(Blockout_d_T_m_SG_D_1_f7f20) -> T_m_SG_D_1/1
  d_Px_2_SG_D_1_block/1(Blockout_d_Px_2_SG_D_1_42534) -> Px_2_SG_D_1/1
  psi_gq_SG_D_1/1 -> d_psi_kq_SG_D_1_block/1(State_psi_gq_SG_D_1_14615), d_psi_kq_SG_D_1_block/3(State_psi_gq_SG_D_1_19905), d_psi_gq_SG_D_1_block/1(State_psi_gq_SG_D_1_779cb), d_psi_gq_SG_D_1_block/2(State_psi_gq_SG_D_1_8746a), d_psi_gq_SG_D_1_block/4(State_psi_gq_SG_D_1_7f7a6), d_psi_gq_SG_D_1_block/7(State_psi_gq_SG_D_1_89958), T_e_SG_D_1_block/2(State_psi_gq_SG_D_1_b4b18), i_q_SG_D_1_block/1(State_psi_gq_SG_D_1_ea88a), i_d_SG_D_1_block/1(State_psi_gq_SG_D_1_16d47), d_w_SG_D_1_block/4(State_psi_gq_SG_D_1_ba39e), d_V_f_SG_D_1_block/9(State_psi_gq_SG_D_1_45243), d_psi_q_SG_D_1_block/1(State_psi_gq_SG_D_1_d2ce1)
  psi_fd_SG_D_1/1 -> i_d_SG_D_1_block/7(State_psi_fd_SG_D_1_32fec), d_w_SG_D_1_block/10(State_psi_fd_SG_D_1_b7bc4), i_q_SG_D_1_block/7(State_psi_fd_SG_D_1_79f47), d_psi_1d_SG_D_1_block/5(State_psi_fd_SG_D_1_eccee), d_psi_1d_SG_D_1_block/2(State_psi_fd_SG_D_1_bca21), T_e_SG_D_1_block/8(State_psi_fd_SG_D_1_1100d), d_V_f_SG_D_1_block/6(State_psi_fd_SG_D_1_16d3d), d_psi_d_SG_D_1_block/3(State_psi_fd_SG_D_1_6e896), d_psi_fd_SG_D_1_block/7(State_psi_fd_SG_D_1_0c561), d_psi_fd_SG_D_1_block/10(State_psi_fd_SG_D_1_ff8b9), d_psi_fd_SG_D_1_block/4(State_psi_fd_SG_D_1_ce065), d_psi_fd_SG_D_1_block/2(State_psi_fd_SG_D_1_70a07)
  d_E_fd_SG_D_1_block/1(Blockout_d_E_fd_SG_D_1_51f8a) -> E_fd_SG_D_1/1
  psi_1d_SG_D_1/1 -> d_psi_fd_SG_D_1_block/8(State_psi_1d_SG_D_1_5c1e0), d_psi_fd_SG_D_1_block/5(State_psi_1d_SG_D_1_745e7), d_psi_fd_SG_D_1_block/3(State_psi_1d_SG_D_1_5420c), d_psi_d_SG_D_1_block/1(State_psi_1d_SG_D_1_86041), d_V_f_SG_D_1_block/4(State_psi_1d_SG_D_1_891e1), d_w_SG_D_1_block/8(State_psi_1d_SG_D_1_e1fe4), i_d_SG_D_1_block/5(State_psi_1d_SG_D_1_2c6db), i_q_SG_D_1_block/5(State_psi_1d_SG_D_1_2130a), d_psi_1d_SG_D_1_block/3(State_psi_1d_SG_D_1_c520a), d_psi_1d_SG_D_1_block/1(State_psi_1d_SG_D_1_d2762), T_e_SG_D_1_block/6(State_psi_1d_SG_D_1_94903)
  Px_2_SG_D_1/1 -> d_Px_3_SG_D_1_block/2(State_Px_2_SG_D_1_7ed7d), d_Px_3_SG_D_1_block/3(State_Px_2_SG_D_1_8a060), d_Px_2_SG_D_1_block/1(State_Px_2_SG_D_1_42d3f)
  T_m_SG_D_1/1 -> d_T_m_SG_D_1_block/2(State_T_m_SG_D_1_00082), d_w_SG_D_1_block/2(State_T_m_SG_D_1_32a5a)
  theta_SG_D_1/1 -> d_psi_d_SG_D_1_block/5(State_theta_SG_D_1_15a2a), d_psi_d_SG_D_1_block/7(State_theta_SG_D_1_2debe), d_psi_q_SG_D_1_block/7(State_theta_SG_D_1_4ed40), d_psi_q_SG_D_1_block/5(State_theta_SG_D_1_ab583), theta_SG_D_1_out_block/1(State_theta_SG_D_1_c9f92), i_q_SG_D_1_block/4(State_theta_SG_D_1_dbec2), i_q_SG_D_1_block/8(State_theta_SG_D_1_fb79e), i_d_SG_D_1_block/4(State_theta_SG_D_1_f0743), i_d_SG_D_1_block/8(State_theta_SG_D_1_03b3d)
  psi_q_SG_D_1/1 -> d_psi_d_SG_D_1_block/8(State_psi_q_SG_D_1_4f741), d_psi_q_SG_D_1_block/3(State_psi_q_SG_D_1_a72f0), d_psi_kq_SG_D_1_block/5(State_psi_q_SG_D_1_673e0), d_psi_gq_SG_D_1_block/6(State_psi_q_SG_D_1_25e6e), d_psi_gq_SG_D_1_block/9(State_psi_q_SG_D_1_d29ab), T_e_SG_D_1_block/4(State_psi_q_SG_D_1_5bbe1), T_e_SG_D_1_block/5(State_psi_q_SG_D_1_be59e), i_q_SG_D_1_block/3(State_psi_q_SG_D_1_2c971), i_d_SG_D_1_block/3(State_psi_q_SG_D_1_6d935), d_w_SG_D_1_block/6(State_psi_q_SG_D_1_5043e), d_w_SG_D_1_block/7(State_psi_q_SG_D_1_624e9), d_V_f_SG_D_1_block/7(State_psi_q_SG_D_1_76896), d_V_f_SG_D_1_block/11(State_psi_q_SG_D_1_a95db)
  v_d_SG_D_1/1 -> d_psi_d_SG_D_1_block/4(Input_v_d_SG_D_1_19f90), d_psi_q_SG_D_1_block/4(Input_v_d_SG_D_1_612c6)
  v_q_SG_D_1/1 -> d_psi_d_SG_D_1_block/6(Input_v_q_SG_D_1_67e4a), d_psi_q_SG_D_1_block/6(Input_v_q_SG_D_1_0e1bb)
  Px_1_SG_D_1/1 -> d_Px_2_SG_D_1_block/3(State_Px_1_SG_D_1_1d3a0), d_Px_2_SG_D_1_block/2(State_Px_1_SG_D_1_862b1), d_Px_3_SG_D_1_block/4(State_Px_1_SG_D_1_12e65), d_Px_3_SG_D_1_block/5(State_Px_1_SG_D_1_8beee), d_Px_1_SG_D_1_block/1(State_Px_1_SG_D_1_0d11e)
  psi_d_SG_D_1/1 -> d_psi_fd_SG_D_1_block/6(State_psi_d_SG_D_1_789f5), d_psi_fd_SG_D_1_block/9(State_psi_d_SG_D_1_61bb9), T_e_SG_D_1_block/1(State_psi_d_SG_D_1_0962a), T_e_SG_D_1_block/7(State_psi_d_SG_D_1_5996b), d_psi_1d_SG_D_1_block/4(State_psi_d_SG_D_1_3f3ac), i_q_SG_D_1_block/6(State_psi_d_SG_D_1_6fa4d), i_d_SG_D_1_block/6(State_psi_d_SG_D_1_87c65), d_w_SG_D_1_block/3(State_psi_d_SG_D_1_67592), d_w_SG_D_1_block/9(State_psi_d_SG_D_1_602b1), d_V_f_SG_D_1_block/5(State_psi_d_SG_D_1_03284), d_V_f_SG_D_1_block/12(State_psi_d_SG_D_1_e5451), d_psi_q_SG_D_1_block/8(State_psi_d_SG_D_1_23bff), d_psi_d_SG_D_1_block/2(State_psi_d_SG_D_1_dbe44)
  d_psi_kq_SG_D_1_block/1(Blockout_d_psi_kq_SG_D_1_42599) -> psi_kq_SG_D_1/1
  d_psi_gq_SG_D_1_block/1(Blockout_d_psi_gq_SG_D_1_50e01) -> psi_gq_SG_D_1/1
  T_e_SG_D_1_block/1(Blockout_T_e_SG_D_1_6e908) -> T_e_SG_D_1/1
  d_psi_1d_SG_D_1_block/1(Blockout_d_psi_1d_SG_D_1_4de60) -> psi_1d_SG_D_1/1
  i_q_SG_D_1_block/1(Blockout_i_q_SG_D_1_e8e0f) -> i_q_SG_D_1/1
  i_d_SG_D_1_block/1(Blockout_i_d_SG_D_1_3e23c) -> i_d_SG_D_1/1
  d_w_SG_D_1_block/1(Blockout_d_w_SG_D_1_21724) -> w_SG_D_1/1
  d_V_f_SG_D_1_block/1(Blockout_d_V_f_SG_D_1_4bc37) -> V_f_SG_D_1/1
  d_R_f_SG_D_1_block/1(Blockout_d_R_f_SG_D_1_13d30) -> R_f_SG_D_1/1
  theta_SG_D_1_out_block/1(Blockout_theta_SG_D_1_out_eb1bc) -> theta_SG_D_1_out/1
  d_psi_q_SG_D_1_block/1(Blockout_d_psi_q_SG_D_1_96a28) -> psi_q_SG_D_1/1
  d_psi_d_SG_D_1_block/1(Blockout_d_psi_d_SG_D_1_534f2) -> psi_d_SG_D_1/1
  R_f_SG_D_1/1 -> d_V_f_SG_D_1_block/2(State_R_f_SG_D_1_d9482), d_R_f_SG_D_1_block/2(State_R_f_SG_D_1_cc465)
  Px_3_SG_D_1/1 -> d_V_f_SG_D_1_block/3(State_Px_3_SG_D_1_ece67), d_Px_3_SG_D_1_block/1(State_Px_3_SG_D_1_8bd18)
  E_fd_SG_D_1/1 -> d_V_f_SG_D_1_block/1(State_E_fd_SG_D_1_d7c8e), d_R_f_SG_D_1_block/1(State_E_fd_SG_D_1_36333), d_psi_fd_SG_D_1_block/1(State_E_fd_SG_D_1_52367), d_E_fd_SG_D_1_block/1(State_E_fd_SG_D_1_82d72)
  d_psi_fd_SG_D_1_block/1(Blockout_d_psi_fd_SG_D_1_0c186) -> psi_fd_SG_D_1/1

== system IEEE9Buses/SG_D_2 ==
  v_d_SG_D_2 : Inport
  v_q_SG_D_2 : Inport  Port=2
  E_fd_SG_D_2 : Integrator  InitialCondition=3.3252622445371984
  Px_1_SG_D_2 : Integrator  InitialCondition=0.0
  Px_2_SG_D_2 : Integrator  InitialCondition=0.0
  Px_3_SG_D_2 : Integrator  InitialCondition=8.772813347812148e-25
  R_f_SG_D_2 : Integrator  InitialCondition=22.450270525261146
  T_e_SG_D_2_block : Subsystem
  T_m_SG_D_2 : Integrator  InitialCondition=1.6329134569704846
  V_f_SG_D_2 : Integrator  InitialCondition=33.25262244537199
  d_E_fd_SG_D_2_block : Subsystem
  d_Px_1_SG_D_2_block : Subsystem
  d_Px_2_SG_D_2_block : Subsystem
  d_Px_3_SG_D_2_block : Subsystem
  d_R_f_SG_D_2_block : Subsystem
  d_T_m_SG_D_2_block : Subsystem
  d_V_f_SG_D_2_block : Subsystem
  d_psi_1d_SG_D_2_block : Subsystem
  d_psi_d_SG_D_2_block : Subsystem
  d_psi_fd_SG_D_2_block : Subsystem
  d_psi_gq_SG_D_2_block : Subsystem
  d_psi_kq_SG_D_2_block : Subsystem
  d_psi_q_SG_D_2_block : Subsystem
  d_theta_SG_D_2_block : Subsystem
  d_w_SG_D_2_block : Subsystem
  i_d_SG_D_2_block : Subsystem
  i_q_SG_D_2_block : Subsystem
  psi_1d_SG_D_2 : Integrator  InitialCondition=0.5649408845898252
  psi_d_SG_D_2 : Integrator  InitialCondition=0.49033760459124737
  psi_fd_SG_D_2 : Integrator  InitialCondition=0.9409414157826567
  psi_gq_SG_D_2 : Integrator  InitialCondition=0.5375796146311603
  psi_kq_SG_D_2 : Integrator  InitialCondition=-0.839968147861188
  psi_q_SG_D_2 : Integrator  InitialCondition=-0.8735668737756356
  theta_SG_D_2 : Integrator  InitialCondition=1.2279092931343085
  theta_SG_D_2_out_block : Subsystem
  w_SG_D_2 : Integrator  InitialCondition=376.99111843077515
  w_SG_D_2_out_block : Subsystem
  i_d_SG_D_2 : Outport
  i_q_SG_D_2 : Outport  Port=2
  T_e_SG_D_2 : Outport  Port=3
  w_SG_D_2_out : Outport  Port=4
  theta_SG_D_2_out : Outport  Port=5
  wires:
  T_e_SG_D_2_block/1(Blockout_T_e_SG_D_2_58459) -> T_e_SG_D_2/1
  d_Px_2_SG_D_2_block/1(Blockout_d_Px_2_SG_D_2_af1ce) -> Px_2_SG_D_2/1
  d_T_m_SG_D_2_block/1(Blockout_d_T_m_SG_D_2_06e02) -> T_m_SG_D_2/1
  w_SG_D_2/1 -> d_w_SG_D_2_block/1(State_w_SG_D_2_206aa), d_psi_q_SG_D_2_block/9(State_w_SG_D_2_3e2aa), d_V_f_SG_D_2_block/8(State_w_SG_D_2_96164), d_V_f_SG_D_2_block/13(State_w_SG_D_2_fc940), d_T_m_SG_D_2_block/1(State_w_SG_D_2_fe2e1), d_theta_SG_D_2_block/1(State_w_SG_D_2_ade08), d_Px_1_SG_D_2_block/2(State_w_SG_D_2_2f75d), d_Px_2_SG_D_2_block/4(State_w_SG_D_2_4c038), d_Px_3_SG_D_2_block/6(State_w_SG_D_2_e3ed6), d_psi_d_SG_D_2_block/9(State_w_SG_D_2_33168), w_SG_D_2_out_block/1(State_w_SG_D_2_7ad77)
  d_Px_3_SG_D_2_block/1(Blockout_d_Px_3_SG_D_2_56385) -> Px_3_SG_D_2/1
  psi_kq_SG_D_2/1 -> d_psi_q_SG_D_2_block/2(State_psi_kq_SG_D_2_534a3), d_psi_gq_SG_D_2_block/3(State_psi_kq_SG_D_2_642d1), d_psi_gq_SG_D_2_block/5(State_psi_kq_SG_D_2_cefa6), d_psi_gq_SG_D_2_block/8(State_psi_kq_SG_D_2_5fe1f), d_psi_kq_SG_D_2_block/4(State_psi_kq_SG_D_2_dff77), d_w_SG_D_2_block/5(State_psi_kq_SG_D_2_36273), i_d_SG_D_2_block/2(State_psi_kq_SG_D_2_eb372), i_q_SG_D_2_block/2(State_psi_kq_SG_D_2_83339), d_V_f_SG_D_2_block/10(State_psi_kq_SG_D_2_ecde5), d_psi_kq_SG_D_2_block/2(State_psi_kq_SG_D_2_3768b), T_e_SG_D_2_block/3(State_psi_kq_SG_D_2_a60cc)
  d_Px_1_SG_D_2_block/1(Blockout_d_Px_1_SG_D_2_5baad) -> Px_1_SG_D_2/1
  d_theta_SG_D_2_block/1(Blockout_d_theta_SG_D_2_0ad08) -> theta_SG_D_2/1
  psi_q_SG_D_2/1 -> d_psi_d_SG_D_2_block/8(State_psi_q_SG_D_2_0c26a), d_psi_q_SG_D_2_block/3(State_psi_q_SG_D_2_db54d), d_psi_gq_SG_D_2_block/6(State_psi_q_SG_D_2_d7c9a), d_psi_gq_SG_D_2_block/9(State_psi_q_SG_D_2_6b756), d_psi_kq_SG_D_2_block/5(State_psi_q_SG_D_2_e662c), d_V_f_SG_D_2_block/11(State_psi_q_SG_D_2_841a6), d_w_SG_D_2_block/6(State_psi_q_SG_D_2_19852), i_d_SG_D_2_block/3(State_psi_q_SG_D_2_21c3a), d_w_SG_D_2_block/7(State_psi_q_SG_D_2_aaa50), i_q_SG_D_2_block/3(State_psi_q_SG_D_2_adea4), d_V_f_SG_D_2_block/7(State_psi_q_SG_D_2_26682), T_e_SG_D_2_block/5(State_psi_q_SG_D_2_3ca84), T_e_SG_D_2_block/4(State_psi_q_SG_D_2_25743)
  w_SG_D_2_out_block/1(Blockout_w_SG_D_2_out_8dce1) -> w_SG_D_2_out/1
  psi_gq_SG_D_2/1 -> d_psi_q_SG_D_2_block/1(State_psi_gq_SG_D_2_3b9dd), d_psi_gq_SG_D_2_block/1(State_psi_gq_SG_D_2_06c2a), d_psi_gq_SG_D_2_block/2(State_psi_gq_SG_D_2_ad233), d_psi_gq_SG_D_2_block/4(State_psi_gq_SG_D_2_ba7d0), d_psi_kq_SG_D_2_block/1(State_psi_gq_SG_D_2_2a2b4), d_w_SG_D_2_block/4(State_psi_gq_SG_D_2_7cf12), d_psi_kq_SG_D_2_block/3(State_psi_gq_SG_D_2_8a6ac), d_V_f_SG_D_2_block/9(State_psi_gq_SG_D_2_865cd), i_d_SG_D_2_block/1(State_psi_gq_SG_D_2_90053), d_psi_gq_SG_D_2_block/7(State_psi_gq_SG_D_2_531c1), T_e_SG_D_2_block/2(State_psi_gq_SG_D_2_ad00d), i_q_SG_D_2_block/1(State_psi_gq_SG_D_2_3847f)
  Px_2_SG_D_2/1 -> d_Px_3_SG_D_2_block/2(State_Px_2_SG_D_2_9f207), d_Px_3_SG_D_2_block/3(State_Px_2_SG_D_2_c3e8f), d_Px_2_SG_D_2_block/1(State_Px_2_SG_D_2_f1aec)
  v_d_SG_D_2/1 -> d_psi_d_SG_D_2_block/4(Input_v_d_SG_D_2_823c1), d_psi_q_SG_D_2_block/4(Input_v_d_SG_D_2_f72d1)
  d_V_f_SG_D_2_block/1(Blockout_d_V_f_SG_D_2_c2dc1) -> V_f_SG_D_2/1
  v_q_SG_D_2/1 -> d_psi_d_SG_D_2_block/6(Input_v_q_SG_D_2_1fb2d), d_psi_q_SG_D_2_block/6(Input_v_q_SG_D_2_1bb17)
  psi_1d_SG_D_2/1 -> d_psi_fd_SG_D_2_block/5(State_psi_1d_SG_D_2_69a8e), d_psi_fd_SG_D_2_block/8(State_psi_1d_SG_D_2_6526c), d_psi_fd_SG_D_2_block/3(State_psi_1d_SG_D_2_ddd99), d_psi_1d_SG_D_2_block/3(State_psi_1d_SG_D_2_eff8f), d_V_f_SG_D_2_block/4(State_psi_1d_SG_D_2_c305a), d_psi_1d_SG_D_2_block/1(State_psi_1d_SG_D_2_680ce), d_psi_d_SG_D_2_block/1(State_psi_1d_SG_D_2_5b4b1), i_q_SG_D_2_block/5(State_psi_1d_SG_D_2_91d23), T_e_SG_D_2_block/6(State_psi_1d_SG_D_2_a239a), d_w_SG_D_2_block/8(State_psi_1d_SG_D_2_e97e7), i_d_SG_D_2_block/5(State_psi_1d_SG_D_2_6831d)
  T_m_SG_D_2/1 -> d_T_m_SG_D_2_block/2(State_T_m_SG_D_2_5de5c), d_w_SG_D_2_block/2(State_T_m_SG_D_2_721fe)
  theta_SG_D_2/1 -> d_psi_d_SG_D_2_block/5(State_theta_SG_D_2_159ac), i_d_SG_D_2_block/4(State_theta_SG_D_2_ad8b9), d_psi_d_SG_D_2_block/7(State_theta_SG_D_2_af1f0), i_q_SG_D_2_block/4(State_theta_SG_D_2_b1bab), d_psi_q_SG_D_2_block/7(State_theta_SG_D_2_9667b), i_q_SG_D_2_block/8(State_theta_SG_D_2_88755), d_psi_q_SG_D_2_block/5(State_theta_SG_D_2_4b6fa), i_d_SG_D_2_block/8(State_theta_SG_D_2_d994c), theta_SG_D_2_out_block/1(State_theta_SG_D_2_4fa63)
  i_d_SG_D_2_block/1(Blockout_i_d_SG_D_2_44cd5) -> i_d_SG_D_2/1
  psi_d_SG_D_2/1 -> d_psi_fd_SG_D_2_block/6(State_psi_d_SG_D_2_a4eb1), d_psi_fd_SG_D_2_block/9(State_psi_d_SG_D_2_1bf37), d_psi_d_SG_D_2_block/2(State_psi_d_SG_D_2_c6699), d_psi_q_SG_D_2_block/8(State_psi_d_SG_D_2_ede2a), d_psi_1d_SG_D_2_block/4(State_psi_d_SG_D_2_8d92a), d_w_SG_D_2_block/9(State_psi_d_SG_D_2_aed2c), d_V_f_SG_D_2_block/5(State_psi_d_SG_D_2_df162), d_V_f_SG_D_2_block/12(State_psi_d_SG_D_2_63914), i_d_SG_D_2_block/6(State_psi_d_SG_D_2_b6ace), T_e_SG_D_2_block/1(State_psi_d_SG_D_2_c06bd), T_e_SG_D_2_block/7(State_psi_d_SG_D_2_23d38), i_q_SG_D_2_block/6(State_psi_d_SG_D_2_186b2), d_w_SG_D_2_block/3(State_psi_d_SG_D_2_7ca90)
  Px_1_SG_D_2/1 -> d_Px_3_SG_D_2_block/4(State_Px_1_SG_D_2_15f5c), d_Px_1_SG_D_2_block/1(State_Px_1_SG_D_2_446b7), d_Px_2_SG_D_2_block/3(State_Px_1_SG_D_2_b0ce9), d_Px_3_SG_D_2_block/5(State_Px_1_SG_D_2_308b2), d_Px_2_SG_D_2_block/2(State_Px_1_SG_D_2_41234)
  psi_fd_SG_D_2/1 -> d_psi_fd_SG_D_2_block/4(State_psi_fd_SG_D_2_ebd42), d_psi_fd_SG_D_2_block/7(State_psi_fd_SG_D_2_d7212), d_psi_fd_SG_D_2_block/10(State_psi_fd_SG_D_2_79a88), d_psi_d_SG_D_2_block/3(State_psi_fd_SG_D_2_fabe7), d_psi_1d_SG_D_2_block/2(State_psi_fd_SG_D_2_d51f2), d_psi_fd_SG_D_2_block/2(State_psi_fd_SG_D_2_7c19b), d_V_f_SG_D_2_block/6(State_psi_fd_SG_D_2_e99d0), d_w_SG_D_2_block/10(State_psi_fd_SG_D_2_06fd5), i_d_SG_D_2_block/7(State_psi_fd_SG_D_2_d29ae), i_q_SG_D_2_block/7(State_psi_fd_SG_D_2_f955d), T_e_SG_D_2_block/8(State_psi_fd_SG_D_2_3f2f2), d_psi_1d_SG_D_2_block/5(State_psi_fd_SG_D_2_13ea5)
  d_psi_kq_SG_D_2_block/1(Blockout_d_psi_kq_SG_D_2_b6d40) -> psi_kq_SG_D_2/1
  R_f_SG_D_2/1 -> d_V_f_SG_D_2_block/2(State_R_f_SG_D_2_01caf), d_R_f_SG_D_2_block/2(State_R_f_SG_D_2_9e0bf)
  theta_SG_D_2_out_block/1(Blockout_theta_SG_D_2_out_702a9) -> theta_SG_D_2_out/1
  d_psi_q_SG_D_2_block/1(Blockout_d_psi_q_SG_D_2_456f3) -> psi_q_SG_D_2/1
  d_psi_1d_SG_D_2_block/1(Blockout_d_psi_1d_SG_D_2_990c9) -> psi_1d_SG_D_2/1
  d_R_f_SG_D_2_block/1(Blockout_d_R_f_SG_D_2_1e3df) -> R_f_SG_D_2/1
  d_w_SG_D_2_block/1(Blockout_d_w_SG_D_2_853c5) -> w_SG_D_2/1
  d_psi_d_SG_D_2_block/1(Blockout_d_psi_d_SG_D_2_d579c) -> psi_d_SG_D_2/1
  d_psi_gq_SG_D_2_block/1(Blockout_d_psi_gq_SG_D_2_fc324) -> psi_gq_SG_D_2/1
  i_q_SG_D_2_block/1(Blockout_i_q_SG_D_2_7be03) -> i_q_SG_D_2/1
  V_f_SG_D_2/1 -> d_E_fd_SG_D_2_block/2(State_V_f_SG_D_2_155d9), d_V_f_SG_D_2_block/14(State_V_f_SG_D_2_5ee1c)
  Px_3_SG_D_2/1 -> d_V_f_SG_D_2_block/3(State_Px_3_SG_D_2_3a89c), d_Px_3_SG_D_2_block/1(State_Px_3_SG_D_2_01548)
  d_E_fd_SG_D_2_block/1(Blockout_d_E_fd_SG_D_2_eb42a) -> E_fd_SG_D_2/1
  E_fd_SG_D_2/1 -> d_V_f_SG_D_2_block/1(State_E_fd_SG_D_2_4b548), d_R_f_SG_D_2_block/1(State_E_fd_SG_D_2_fa033), d_E_fd_SG_D_2_block/1(State_E_fd_SG_D_2_bb78e), d_psi_fd_SG_D_2_block/1(State_E_fd_SG_D_2_4ddbc)
  d_psi_fd_SG_D_2_block/1(Blockout_d_psi_fd_SG_D_2_e3965) -> psi_fd_SG_D_2/1
